simulink subsystem "DelfiaBoatWithController"  (R2020b)
settings: Solver=VariableStepAuto  StartTime=0.0  StopTime=10.0  RelTol=1e-3
undefined symbols (not defined in the file or in its folder): d11, d22, d23, d32, d33, I, m
settings Model: Creator=boers  LastModifiedBy=boers

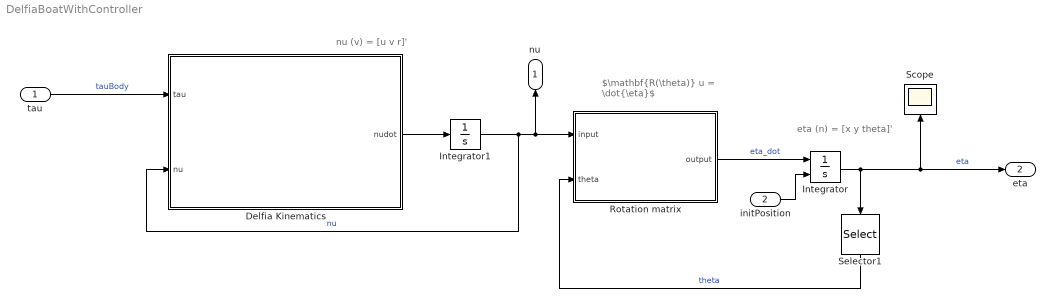
== system DelfiaBoatWithController ==
  note: eta (n) = [x y theta]'
  note: $\mathbf{R(\theta)}\nu = \dot{\eta}$
  note: nu (v) = [u v r]'
  tau : Inport
  initPosition : Inport  Port=2
  Delfia Kinematics : Subsystem
  Integrator : Integrator  InitialConditionSource=external  InitialCondition=[0 0 pi/4]
  Integrator1 : Integrator  InitialCondition=[0 0 0]
  Rotation matrix : MATLAB Function  TreatAsAtomicUnit=on
  Scope : Scope
  Selector1 : Selector  InputPortWidth=3  IndexOptions=Index vector (dialog)  Indices=[3]  OutputSizes=1
  nu : Outport
  eta : Outport  Port=2
  wires:
  Rotation matrix/1(output) -> Integrator/1  "eta_dot"
  Integrator/1 -> Selector1/1, Scope/1, eta/1  "eta"
  Integrator1/1 -> Delfia Kinematics/2(nu), nu/1, Rotation matrix/1(input)  "nu"
  tau/1 -> Delfia Kinematics/1(tau)  "tauBody"
  Selector1/1 -> Rotation matrix/2(theta)  "theta"
  Delfia Kinematics/1(nudot) -> Integrator1/1
  initPosition/1 -> Integrator/2

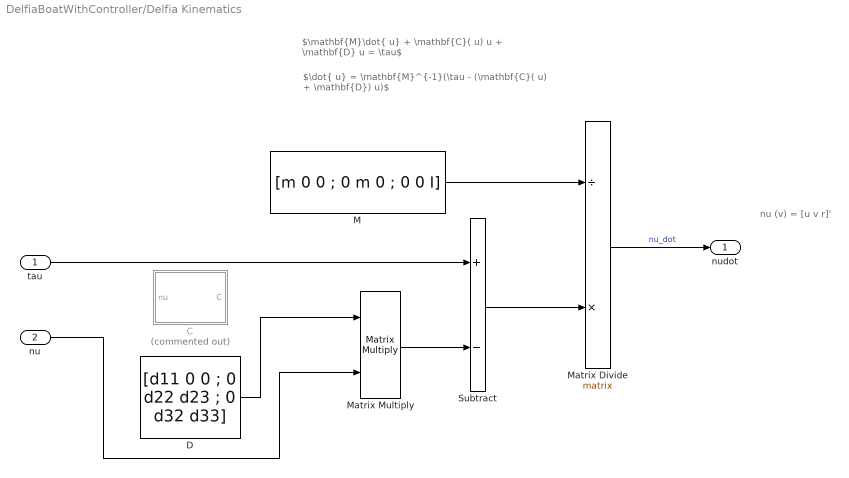
== system DelfiaBoatWithController/Delfia Kinematics ==
  note: $\dot{\nu} = \mathbf{M}^{-1}(\tau - (\mathbf{C}(\nu) + \mathbf{D})\nu)$
  note: $\mathbf{M}\dot{\nu} + \mathbf{C}(\nu)\nu + \mathbf{D}\nu = \tau$
  note: nu (v) = [u v r]'
  tau : Inport
  nu : Inport  Port=2
  C : MATLAB Function  Commented=on  TreatAsAtomicUnit=on
  D : Constant  Value=[d11 0 0 ; 0 d22 d23 ; 0 d32 d33]
  M : Constant  Value=[m 0 0 ; 0 m 0 ; 0 0 I]
  Matrix Divide : Product  Inputs=/*  Multiplication=Matrix(*)
  Matrix Multiply : Product  Multiplication=Matrix(*)
  Subtract : Sum  Inputs=+-
  nudot : Outport
  wires:
  nu/1 -> Matrix Multiply/2
  tau/1 -> Subtract/1
  Subtract/1 -> Matrix Divide/2
  Matrix Divide/1 -> nudot/1  "nu_dot"
  D/1 -> Matrix Multiply/1
  M/1 -> Matrix Divide/1
  Matrix Multiply/1 -> Subtract/2

== matlab function DelfiaBoatWithController/Rotation matrix ==
  data: input input; output output; theta input
function output = BodyToGlobal(input, theta)

rotation_matrix =  [cos(theta) -sin(theta) 0;
                    sin(theta)  cos(theta) 0;
                            0           0  1];

output = rotation_matrix * input;

== matlab function DelfiaBoatWithController/Delfia Kinematics/C ==
  data: nu input; C output
function C = fcn(nu)

m = 3.345; %[Kg]     
I = 0.031; %[Kg · m2]
d11 = 2.7343;        
d22 = 4.6025;        
d23 = 0.0;       
d32 = 0.0;       
d33 = 0.22243;       
Xudot = 0.2310;      
Yvdot = 1.334;       
Yrdot = 0;           
Nrdot = 0.110; 


u = nu(1);
v = nu(2);
r = nu(3);

Crb = [0    0   -m*v;
       0    0   m*u ;
       m*v -m*u   0 ];

Ca = [0                     0            Yvdot*v + Yrdot*r;
      0                     0           -Xudot*u          ;
      -Yvdot*v + Yrdot*r    Xudot*u     0                 ];

C = Crb + Ca;
